simulink model "Three_Phase6PulseRectifier"  (R2025a)
settings: Solver=VariableStepAuto  StartTime=0.0  StopTime=1  RelTol=1e-3
libraries: spsDiodeLib x6, spsVoltageMeasurementLib x4, spsACVoltageSourceLib x3, spsCurrentMeasurementLib x3, spsGroundLib x1, spsSeriesRLCBranchLib x1, sps_lib x1
settings Model: LastModifiedBy=jaivi

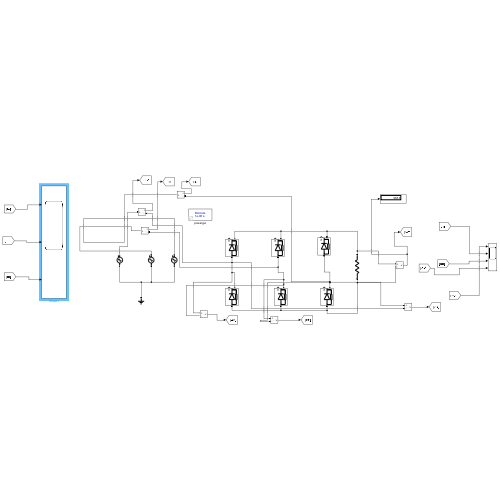
[thumbnail: Simulink's stored preview of the top-level diagram]
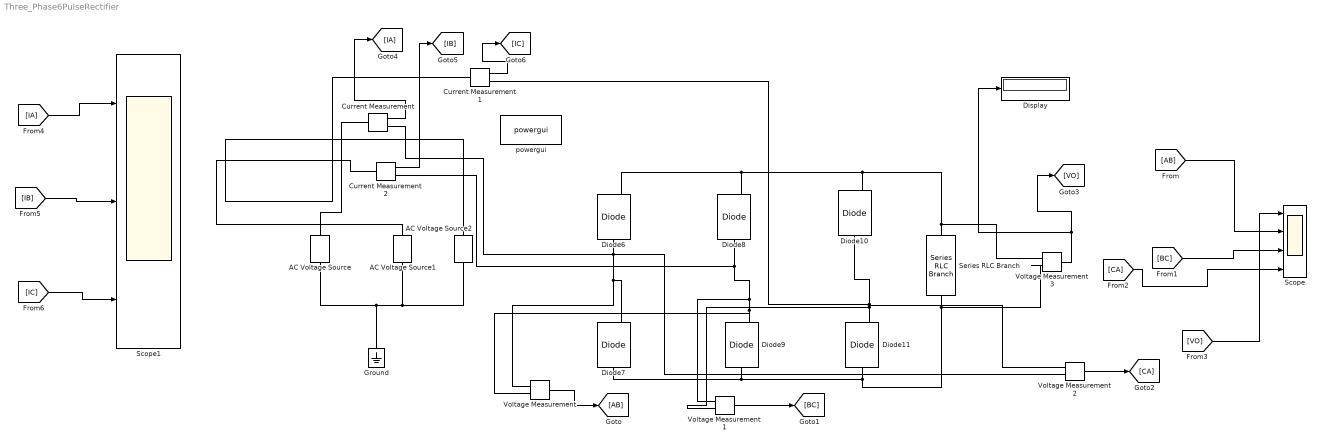
== system Three_Phase6PulseRectifier ==
  AC Voltage Source : spsACVoltageSourceLib/AC Voltage Source  Amplitude=254  Phase=0  Frequency=50  SampleTime=0  Measurements=None  BusType=swing  Pref=10e3  Qref=0  Qmin=-inf  Qmax=+inf
  AC Voltage Source1 : spsACVoltageSourceLib/AC Voltage Source  Amplitude=254  Phase=120  Frequency=50  SampleTime=0  Measurements=None  BusType=swing  Pref=10e3  Qref=0  Qmin=-inf  Qmax=+inf
  AC Voltage Source2 : spsACVoltageSourceLib/AC Voltage Source  Amplitude=254  Phase=-120  Frequency=50  SampleTime=0  Measurements=None  BusType=swing  Pref=10e3  Qref=0  Qmin=-inf  Qmax=+inf
  Current Measurement : spsCurrentMeasurementLib/Current Measurement  PhasorSimulation=off  OutputType=Complex  PSBequivalent=0
  Current Measurement1 : spsCurrentMeasurementLib/Current Measurement  PhasorSimulation=off  OutputType=Complex  PSBequivalent=0
  Current Measurement2 : spsCurrentMeasurementLib/Current Measurement  PhasorSimulation=off  OutputType=Complex  PSBequivalent=0
  Diode{6..11} (6 alike) : spsDiodeLib/Diode  Ron=0.001  Lon=0  Vf=0.8  IC=0  UseSnubber=0  Rs=500  Cs=250e-9  Measurements=on
  Display : Display
  Ground : spsGroundLib/Ground  LConnTagsString=a
  Scope : Scope  NumInputPorts=4
      settings: ActiveDisplayYMinimum=367.35199365909091  ActiveDisplayYMaximum=462.02348232386367
  Scope1 : Scope  NumInputPorts=3
      settings: ActiveDisplayYMinimum=-9.3709779515424  ActiveDisplayYMaximum=11.063027664589793  DataLoggingVariableName=ia
  Series RLC Branch : spsSeriesRLCBranchLib/Series RLC Branch  LConnTagsString=__new0  RConnTagsString=__new0  BranchType=R  Resistance=100  Inductance=0  SetiL0=off  InitialCurrent=0  Capacitance=0  Setx0=off  InitialVoltage=0  Measurements=None
  Voltage Measurement : spsVoltageMeasurementLib/Voltage Measurement  Tag=Vab  PhasorSimulation=off  OutputType=Complex  PSBequivalent=0
  Voltage Measurement1 : spsVoltageMeasurementLib/Voltage Measurement  PhasorSimulation=off  OutputType=Complex  PSBequivalent=0
  Voltage Measurement2 : spsVoltageMeasurementLib/Voltage Measurement  PhasorSimulation=off  OutputType=Complex  PSBequivalent=0
  Voltage Measurement3 : spsVoltageMeasurementLib/Voltage Measurement  PhasorSimulation=off  OutputType=Complex  PSBequivalent=0
  powergui : sps_lib/powergui  Priority=1  SimulationMode=Discrete  SampleTime=1e-6  frequency=60  Iterations=50  frequencyindice=50  Pbase=100e6  ErrMax=1e-4  UnitsV=kV  UnitsW=MW  buscounter=0  FunctionMessages=off  echomessages=off  EnableUseOfTLC=off  CurrentSourceSwitches=off  DisableSnubberDevices=off  DisableRonSwitches=off  DisableVfSwitches=off  DisplayEquations=off  AutomaticDiscreteSolvers=off  SolverType=Tustin/Backward Euler (TBE)  Interpol=off  ExternalGateDelay=off  methode=off  Ts=100  x0status=blocks  SPID=on  SwTol=0  HookPort=off  NonlinearTolerance=1e-4  nMaxIteration=100  ContinueOnMaxIteration=off  RestoreLinks=warning  ResistiveCurrentMeasurement=off  Frange=[0:2:500]  Ylog=off  Xlog=on  ShowGrid=off  save=off  variable=ZData  structure=0  ZoomFFT=off  StartTime=0.0  cycles=1  DisplayStyle=1  fundamental=60  FreqAxis=off  MaxFrequency=1000  frequencyindicesteady=1  RmsSteady=1  display=off
  wires:
  Voltage Measurement/1 -> [AB]
  Voltage Measurement1/1 -> [BC]
  Voltage Measurement2/1 -> [CA]
  [AB] -> Scope/2
  Voltage Measurement3/1 -> Display/1, [VO]
  [VO] -> Scope/1
  [BC] -> Scope/3
  [CA] -> Scope/4
  Current Measurement/1 -> [IA]
  Current Measurement2/1 -> [IB]
  Current Measurement1/1 -> [IC]
  [IA] -> Scope1/1
  [IB] -> Scope1/2
  [IC] -> Scope1/3
  connections:
  Series RLC Branch/RConn1 -- Diode11/LConn1 -- Diode9/LConn1 -- Diode7/LConn1 -- Voltage Measurement3/LConn2
  Diode7/RConn1 -- Current Measurement/RConn1 -- Voltage Measurement2/LConn2 -- Diode6/LConn1 -- Voltage Measurement/LConn1
  Diode9/RConn1 -- Voltage Measurement1/LConn1 -- Current Measurement2/RConn1 -- Diode8/LConn1 -- Voltage Measurement/LConn2
  Diode11/RConn1 -- Current Measurement1/RConn1 -- Diode10/LConn1 -- Voltage Measurement2/LConn1 -- Voltage Measurement1/LConn2
  Diode10/RConn1 -- Diode6/RConn1 -- Diode8/RConn1 -- Voltage Measurement3/LConn1 -- Series RLC Branch/LConn1
  Ground/LConn1 -- AC Voltage Source/LConn1 -- AC Voltage Source1/LConn1 -- AC Voltage Source2/LConn1
  AC Voltage Source/RConn1 -- Current Measurement/LConn1
  Current Measurement2/LConn1 -- AC Voltage Source1/RConn1
  Current Measurement1/LConn1 -- AC Voltage Source2/RConn1
